simulink model "fcn"  (Simulink 7.6)
settings: Solver=ode3  StartTime=0.0  StopTime=10.0  FixedStep=1  RelTol=1e-3
settings Model: Creator=hnine  LastModifiedBy=c2wt
settings OptimizationCC: InitFltsAndDblsToZero=on
settings DebuggingCC: SaveWithParameterizedLinksMsg=none  StrictBusMsg=Warning
settings SFSimCC: SimParseCustomCode=off
settings GRTTargetCC: TargetFcnLib=ansi_tfl_tmw.mat

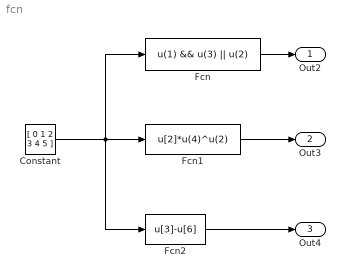
== system fcn ==
  Constant : Constant  Value=[ 0 1 2 3 4 5 ]  VectorParams1D=off
  Fcn : Fcn  Expr=u(1) && u(3) || u(2)
  Fcn1 : Fcn  Expr=u[2]*u(4)^u(2)
  Fcn2 : Fcn  Expr=u[3]-u[6]
  Out2 : Outport
  Out3 : Outport  Port=2
  Out4 : Outport  Port=3
  wires:
  Constant/1 -> Fcn/1, Fcn1/1, Fcn2/1
  Fcn/1 -> Out2/1
  Fcn1/1 -> Out3/1
  Fcn2/1 -> Out4/1
